simulink model "formationFlightSimulation"  (R2024b)
settings: Solver=VariableStepAuto  StartTime=0.0  StopTime=10  RelTol=1e-3
values from neighbouring files (symbols this model uses):
  initialState = zeros(numUAVs*8,1)    [exampleHelperMultiUAVSetupScript.m]
undefined symbols (not defined in the file or in its folder): numUAVs
libraries: uavutilslib x1
settings Model: DataDictionary=formationFlightSimulationData.sldd  Creator=The MathWorks, Inc.  LastModifiedBy=The MathWorks, Inc.

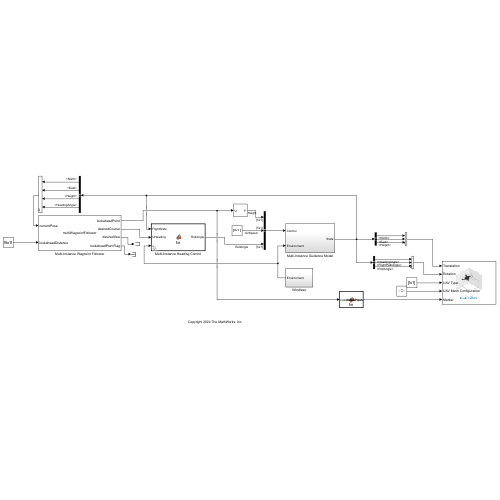
[thumbnail: Simulink's stored preview of the top-level diagram]
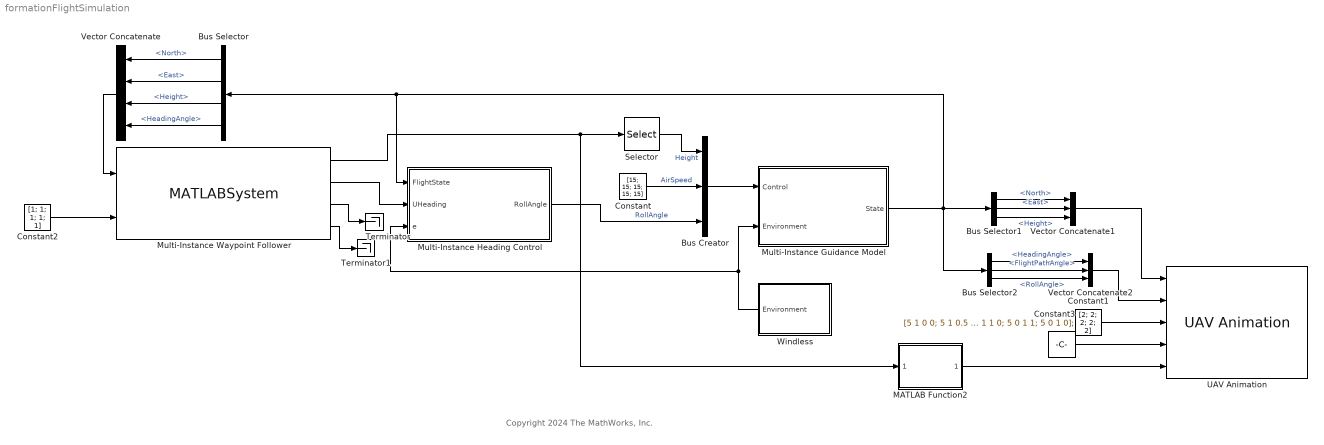
== system formationFlightSimulation ==
  note: Copyright 2024 The MathWorks, Inc.
  Bus Creator : BusCreator  Inputs=3  OutDataTypeStr=Bus: MultiFixedWingControlBus  NonVirtualBus=on
  Bus Selector : BusSelector  OutputSignals=North,East,Height,HeadingAngle
  Bus Selector1 : BusSelector  OutputSignals=North,East,Height
  Bus Selector2 : BusSelector  OutputSignals=HeadingAngle,FlightPathAngle,RollAngle
  Constant : Constant  Value=[15; 15; 15; 15; 15]
  Constant1 : Constant  Value=[2; 2; 2; 2; 2]  VectorParams1D=off
  Constant2 : Constant  Value=[1; 1; 1; 1; 1]
  Constant3 : Constant  Value=[5 1 0 0; 5 1 0.5 1; 5 1 1 0; 5 0 1 1; 5 0 1 0];  VectorParams1D=off
  MATLAB Function2 : MATLAB Function  TreatAsAtomicUnit=on
  Multi-Instance Guidance Model : Subsystem
  Multi-Instance Heading Control : MATLAB Function  TreatAsAtomicUnit=on  mask{numInstanc=numUAVs, PHeadingAngle=0.8}
      mask prompts: numInstanc "Number of instances"; PHeadingAngle "Heading Angle Control Gain"
  Multi-Instance Waypoint Follower : MATLABSystem  System=multiWaypointFollower  MaxFollowers=100  NumUAVs=numUAVs  UAVType={'fixed-wing', 'fixed-wing', 'fixed-wing', 'fixed-wing', 'fixed-wing'}  StartsFrom={'first', 'first', 'first', 'first', 'first'}  TransitionRadiusSource={'internal', 'internal', 'internal', 'internal', 'internal'}  TransitionRadius=[10 10 10 10 10]  MinimumLookaheadDistance=[0.1 0.1 0.1 0.1 0.1]  Waypoints=wayPoints
      mask Type: multiWaypointFollower
      mask Display:
      | disp('multiWaypointFollower');
      | port_label('input',1,'currentPose');
      | port_label('input',2,'lookaheadDistance');
      | port_label('output',1,'lookaheadPoint');
      | port_label('output',2,'desiredCourse');
      | port_label('output',3,'desiredYaw');
      | port_label('output',4,'lookaheadPointFlag');
  Selector : Selector  NumberOfDimensions=2  InputPortWidth=3  IndexOptions=Select all,Index vector (dialog)  Indices=[1 3],3  OutputSizes=1,1
  Terminator : Terminator
  Terminator1 : Terminator
  UAV Animation : uavutilslib/UAV Animation  NumUAV=numUAVs  DynamicUAVConfig=on  UAVType=Multirotor  UAVSize=1  UAVColor=[1 0 0]  UAVTrajectoryAlpha=1  InertialZDirection=Down  RotationFormat=Euler ZYX  DrawMarkers=on  SampleTime=-1
  Vector Concatenate : Concatenate  NumInputs=4  Mode=Multidimensional array  ConcatenateDimension=2
  Vector Concatenate1 : Concatenate  NumInputs=3  Mode=Multidimensional array  ConcatenateDimension=2
  Vector Concatenate2 : Concatenate  NumInputs=3  Mode=Multidimensional array  ConcatenateDimension=2
  Windless : Subsystem  VariantControl=NoWind
  wires:
  Multi-Instance Waypoint Follower/2 -> Multi-Instance Heading Control/2(UHeading)
  Multi-Instance Waypoint Follower/3 -> Terminator/1
  Multi-Instance Waypoint Follower/4 -> Terminator1/1
  Multi-Instance Waypoint Follower/1 -> Selector/1, MATLAB Function2/1(lookAheadPoints)
  Selector/1 -> Bus Creator/1  "Height"
  Multi-Instance Heading Control/1(RollAngle) -> Bus Creator/3  "RollAngle"
  Constant/1 -> Bus Creator/2  "AirSpeed"
  Bus Creator/1 -> Multi-Instance Guidance Model/1(Control)
  Windless/1(Environment) -> Multi-Instance Guidance Model/2(Environment), Multi-Instance Heading Control/3(e)
  Multi-Instance Guidance Model/1(State) -> Bus Selector1/1, Bus Selector2/1, Multi-Instance Heading Control/1(FlightState), Bus Selector/1
  Constant2/1 -> Multi-Instance Waypoint Follower/2
  Bus Selector/1 -> Vector Concatenate/1  "<North>"
  Bus Selector/2 -> Vector Concatenate/2  "<East>"
  Bus Selector/3 -> Vector Concatenate/3  "<Height>"
  Bus Selector/4 -> Vector Concatenate/4  "<HeadingAngle>"
  Vector Concatenate/1 -> Multi-Instance Waypoint Follower/1
  Vector Concatenate1/1 -> UAV Animation/1
  Bus Selector1/1 -> Vector Concatenate1/1  "<North>"
  Bus Selector1/2 -> Vector Concatenate1/2  "<East>"
  Bus Selector1/3 -> Vector Concatenate1/3  "<Height>"
  Vector Concatenate2/1 -> UAV Animation/2
  Bus Selector2/1 -> Vector Concatenate2/1  "<HeadingAngle>"
  Bus Selector2/2 -> Vector Concatenate2/2  "<FlightPathAngle>"
  Bus Selector2/3 -> Vector Concatenate2/3  "<RollAngle>"
  MATLAB Function2/1(markerInput) -> UAV Animation/5
  Constant1/1 -> UAV Animation/3
  Constant3/1 -> UAV Animation/4

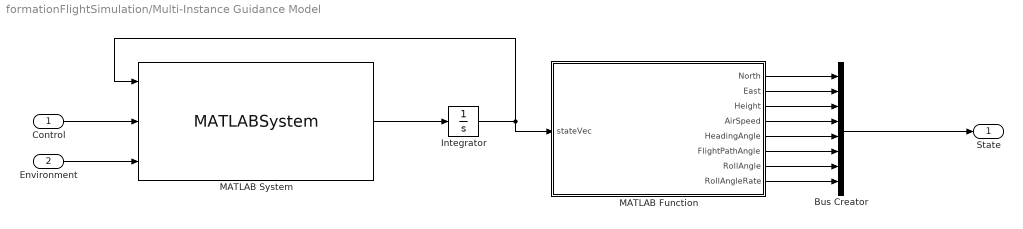
== system formationFlightSimulation/Multi-Instance Guidance Model ==
  Control : Inport
  Environment : Inport  Port=2
  Bus Creator : BusCreator  Inputs=8  OutDataTypeStr=Bus: MultiFixedWingStateBus
  Integrator : Integrator  InitialCondition=initialState
  MATLAB Function : MATLAB Function  TreatAsAtomicUnit=on  mask{numInstances=numUAVs}
      mask prompts: numInstances "Number of instances"
  MATLAB System : MATLABSystem  System=multiFixedwingDerivative  MaxGuidanceModels=100  NumUAVs=numUAVs  Configuration_PDRoll=PDRoll  Configuration_PHeight=PHeight  Configuration_PFlightPathAngle=PFlightPathAngle  Configuration_PAirSpeed=PAirSpeed  Configuration_FlightPathAngleLimits=FlightPathAngleLimits
      mask Type: multiFixedwingDerivative
      mask Display:
      | disp('multiFixedwingDerivative');
      | port_label('input',1,'state');
      | port_label('input',2,'control');
      | port_label('input',3,'env');
      | port_label('output',1,'deriv');
  State : Outport  OutDataTypeStr=Bus: MultiFixedWingStateBus
  wires:
  Control/1 -> MATLAB System/2
  Environment/1 -> MATLAB System/3
  MATLAB System/1 -> Integrator/1
  Integrator/1 -> MATLAB System/1, MATLAB Function/1(stateVec)
  MATLAB Function/1(North) -> Bus Creator/1
  MATLAB Function/2(East) -> Bus Creator/2
  MATLAB Function/3(Height) -> Bus Creator/3
  MATLAB Function/4(AirSpeed) -> Bus Creator/4
  MATLAB Function/5(HeadingAngle) -> Bus Creator/5
  MATLAB Function/6(FlightPathAngle) -> Bus Creator/6
  MATLAB Function/7(RollAngle) -> Bus Creator/7
  MATLAB Function/8(RollAngleRate) -> Bus Creator/8
  Bus Creator/1 -> State/1

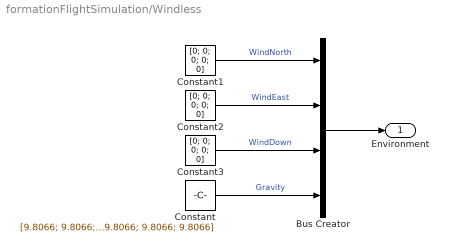
== system formationFlightSimulation/Windless ==
  Bus Creator : BusCreator  Inputs=4  OutDataTypeStr=Bus: MultiFixedWingEnvironmentBus  NonVirtualBus=on
  Constant : Constant  Value=[9.8066; 9.8066; 9.8066; 9.8066; 9.8066]  VectorParams1D=off
  Constant1 : Constant  Value=[0; 0; 0; 0; 0]  VectorParams1D=off
  Constant2 : Constant  Value=[0; 0; 0; 0; 0]  VectorParams1D=off
  Constant3 : Constant  Value=[0; 0; 0; 0; 0]  VectorParams1D=off
  Environment : Outport  VectorParamsAs1DForOutWhenUnconnected=off
  wires:
  Constant2/1 -> Bus Creator/2  "WindEast"
  Constant3/1 -> Bus Creator/3  "WindDown"
  Constant1/1 -> Bus Creator/1  "WindNorth"
  Bus Creator/1 -> Environment/1
  Constant/1 -> Bus Creator/4  "Gravity"

== matlab function formationFlightSimulation/Multi-Instance Guidance Model/MATLAB Function ==
  data: stateVec input; North output; East output; Height output; AirSpeed output; HeadingAngle output; FlightPathAngle output; RollAngle output; RollAngleRate output; numUAVs parameter
function [North, East, Height, AirSpeed, HeadingAngle, FlightPathAngle, RollAngle, RollAngleRate] = vector2struct(stateVec, numUAVs)
    North = zeros(numUAVs,1);
    East = zeros(numUAVs,1);
    Height = zeros(numUAVs,1);
    AirSpeed = zeros(numUAVs,1);
    HeadingAngle = zeros(numUAVs,1);
    FlightPathAngle = zeros(numUAVs,1);
    RollAngle = zeros(numUAVs,1);
    RollAngleRate = zeros(numUAVs,1);

    for i = 1:numUAVs
        North(i) = stateVec((i-1)*8 + 1);
        East(i) = stateVec((i-1)*8 + 2);
        Height(i) = stateVec((i-1)*8 + 3);
        AirSpeed(i) = stateVec((i-1)*8 + 4);
        HeadingAngle(i) = stateVec((i-1)*8 + 5);
        FlightPathAngle(i) = stateVec((i-1)*8 + 6);
        RollAngle(i) = stateVec((i-1)*8 + 7);
        RollAngleRate(i) = stateVec((i-1)*8 + 8);
    end

    
end

== matlab function formationFlightSimulation/Multi-Instance Heading Control ==
  data: FlightState input; RollAngle output; UHeading input; e input; numUAVs parameter; PHeadingAngle parameter
function RollAngle = fcn(FlightState, UHeading, e, numUAVs, PHeadingAngle)
    RollAngle = zeros(numUAVs, 1);
    for i=1:numUAVs
        Va = FlightState.AirSpeed(i);
        HeadingAngle = FlightState.HeadingAngle(i);
        FlightPathAngle = FlightState.FlightPathAngle(i);
        
        YawAngle = HeadingAngle - asin((1/Va)*[e.WindNorth(i), e.WindEast(i)]*[-sin(HeadingAngle); cos(HeadingAngle)]);
        b = [cos(HeadingAngle)*cos(FlightPathAngle), sin(HeadingAngle)*cos(FlightPathAngle), -sin(FlightPathAngle)]*[e.WindNorth(i); e.WindEast(i); e.WindDown(i)];
        c = [e.WindNorth(i), e.WindEast(i), e.WindDown(i)]*[e.WindNorth(i); e.WindEast(i); e.WindDown(i)]- Va^2;
        Vg = -b+sqrt(b^2-c);
        
        RollAngle(i) = atan2(PHeadingAngle*angdiff(HeadingAngle,UHeading(i))*Vg,e.Gravity(i)*cos(HeadingAngle-YawAngle));
    end
    
end

== matlab function formationFlightSimulation/MATLAB Function2 ==
  data: lookAheadPoints input; markerInput output; wayPoints parameter
function markerInput = fcn(lookAheadPoints, wayPoints)

    numUAVs = size(wayPoints, 3);
    numWayPoints = size(wayPoints, 1);

    markerInput = zeros(numWayPoints*numUAVs + numUAVs, 7);
    
    colorArr = [1 0 0; 1 0.5 1; 1 1 0; 0 1 1; 0 1 0];
    for i=1:numUAVs
        markerInput((i-1)*numWayPoints+1: i*numWayPoints,1:3) = wayPoints(:,:,i); % Waypoints position
        markerInput((i-1)*numWayPoints+1: i*numWayPoints,4) = repmat(50,numWayPoints,1); % Waypoints size
        markerInput((i-1)*numWayPoints+1: i*numWayPoints,5:7) = repmat(colorArr(i,:),numWayPoints,1); % Waypoints color (unique for each UAV)
    end

    markerInput(numWayPoints*numUAVs+1:numWayPoints*numUAVs + numUAVs,1:3) = lookAheadPoints(:,:);
    
    for i=1:numUAVs
        markerInput(numWayPoints*numUAVs+i,4) = 50;
        markerInput(numWayPoints*numUAVs+i,5:7) = [0 0 1];
    end
end
